simulink model "Lab7"  (R2021b)
settings: Solver=VariableStepAuto  StartTime=0.0  StopTime=T  RelTol=1e-3
values from neighbouring files (symbols this model uses):
  a = 1/( 2/norm(r0) - dot(v0,v0)/mu_E )    [Excercise1_2223.m]    (also in Excercise2_2223.m; Lab08_script.m = 42164; Lab7_script.m = 16733.65; Lab7_scriptscalar.m = 16733.65)
  A0 = eye(3)    [Lab08_script.m]    (also in Lab7_script.m; Lab7_scriptscalar.m; Lab_GG.m)
  Area_mb = diag([A1 A2 A3 A4 A5 A6])    [Lab08_script.m]    (also in Lab7_script.m)
  e = horizonsresults(:,2)    [Ex3-5.m]    (also in Excercise1_2223.m = 1/mu_E*cross(v,h)-r./vecnorm(r,2,2); Lab08_script.m = 0; Lab7_script.m = 0.1976; Lab7_scriptscalar.m = 0.1976)
  epsilon = (vecnorm(v,2,2)).^2/2-mu_E./vecnorm(r,2,2)    [Excercise1_2223.m]    (also in Lab08_script.m = deg2rad(23.45); Lab7_script.m = deg2rad(23.45); Lab7_scriptscalar.m = deg2rad(23.45))
  I = [Ix 0 0; 0 Iy 0; 0 0 Iz]    [Lab08_script.m]    (also in Lab7_script.m; Lab7_scriptscalar.m; Lab_GG.m)
  i = horizonsresults(:,3)    [Ex3-5.m]    (also in Lab08_script.m = deg2rad(0); Lab7_script.m = deg2rad(60); Lab7_scriptscalar.m = deg2rad(60); ex3_Lambert.m = kep_arr_M(3))
  I_inv = inv(I)    [Lab08_script.m]    (also in Lab7_script.m; Lab7_scriptscalar.m; Lab_GG.m)
  n = 10    [Chapter3.m]    (also in Lab08_script.m = sqrt(mu_E/(a^3)); Lab7_script.m = sqrt(mu_E/(a^3)); Lab7_scriptscalar.m = sqrt(mu_E/(a^3)); Lab_GG.m = sqrt(mu_E/( R_E+r_orbit)^3))
  N_b_mb = [n1'; n2'; n3'; n4'; n5'; n6']    [Lab08_script.m]    (also in Lab7_script.m)
  n_sun = 2*pi/T_sun    (= 1.99238499086e-07)    [Lab08_script.m]    (also in Lab7_script.m; Lab7_scriptscalar.m)
  P = Fe/c    (= 4.52666666667e-06)    [Lab08_script.m]    (also in Lab7_script.m; Lab7_scriptscalar.m)
  rho_d_mb = 0.1    [Lab08_script.m]    (also in Lab7_script.m; Lab7_scriptscalar.m)
  rho_s_mb = 0.5    [Lab08_script.m]    (also in Lab7_script.m; Lab7_scriptscalar.m)
  Rs = astroConstants(2)    [Lab08_script.m]    (also in Lab7_script.m; Lab7_scriptscalar.m)
  theta0 = deg2rad(0)    [Lab08_script.m]    (also in Lab7_script.m = deg2rad(230); Lab7_scriptscalar.m = deg2rad(230))
  v1 = [Y1(:,4) Y1(:,5) Y1(:,6)]    [Excercise2_2223.m]    (also in Lab08_script.m = [0 1 -1]'; Lab7_script.m = [0 1 -1]'; Lab7_scriptscalar.m = [0 1 -1]'; Lab_GG.m = [0 1 -1]')
  v2 = [Y2(:,4) Y2(:,5) Y2(:,6)]    [Excercise2_2223.m]    (also in Lab08_script.m = [-1 0 1]'; Lab7_script.m = [-1 0 1]'; Lab7_scriptscalar.m = [-1 0 1]'; Lab_GG.m = [-1 0 1]')
  v3 = [1 -1 0]'    [Lab08_script.m]    (also in Lab7_script.m; Lab7_scriptscalar.m; Lab_GG.m)
  w_0 = [wx_0 wy_0 wz_0]'    [Lab08_script.m]    (also in Lab7_script.m; Lab7_scriptscalar.m; Lab_GG.m)
libraries: matrix_library x1
settings Model: Creator=sferl  LastModifiedBy=sferl

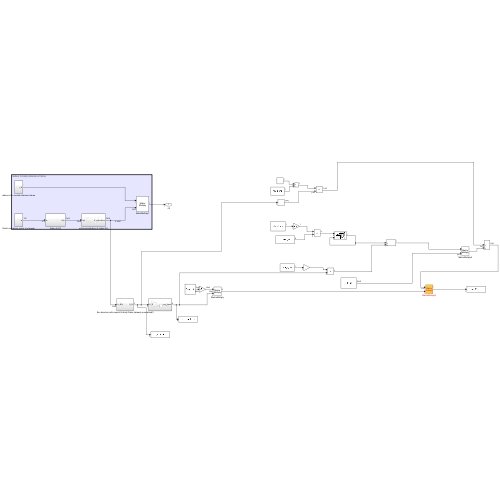
[thumbnail: Simulink's stored preview of the top-level diagram]
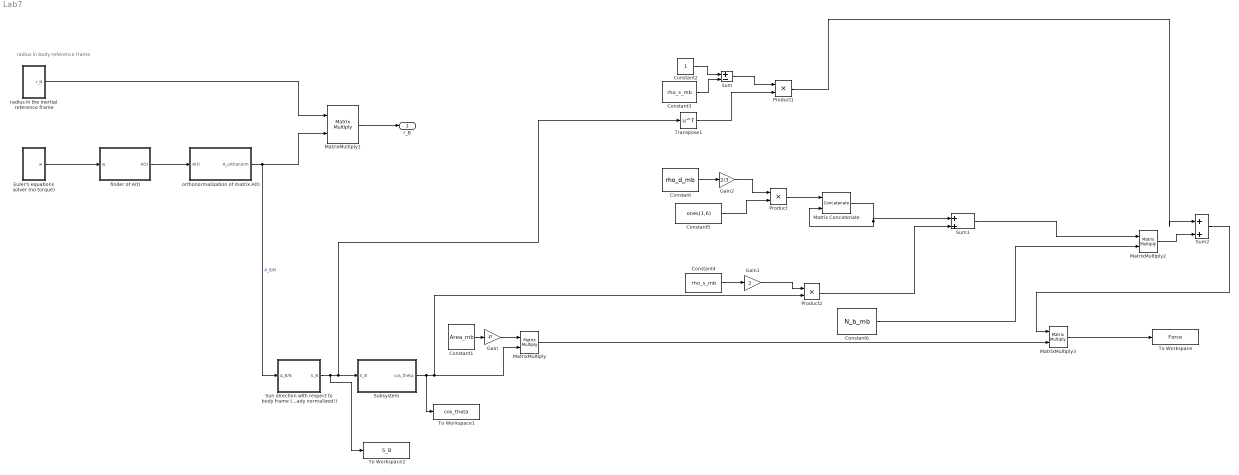
== system Lab7 ==
  note: radius in body reference frame
  Constant : Constant  Value=rho_d_mb
  Constant1 : Constant  Value=Area_mb
  Constant2 : Constant
  Constant3 : Constant  Value=rho_s_mb
  Constant4 : Constant  Value=rho_s_mb
  Constant5 : Constant  Value=ones(1,6)
  Constant6 : Constant  Value=N_b_mb
  Euler's equations solver (no torque) : Subsystem
  Gain : Gain  Gain=-P
  Gain1 : Gain  Gain=2
  Gain2 : Gain  Gain=2/3
  Matrix Concatenate : Concatenate  Mode=Multidimensional array
  MatrixMultiply{,1..3} (4 alike) : Product  Multiplication=Matrix(*)
  Product : Product
  Product1 : Product
  Product2 : Product
  Subsystem : Subsystem
  Sum : Sum  Inputs=+-
  Sum1 : Sum  Inputs=|++
  Sum2 : Sum  Inputs=|++
  Sun direction with respect to body frame (already normalized!) : Subsystem
  To Workspace : ToWorkspace  VariableName=Force  SaveFormat=Timeseries  SampleTime=-1
  To Workspace1 : ToWorkspace  VariableName=cos_theta  SampleTime=-1
  To Workspace2 : ToWorkspace  VariableName=S_B  SampleTime=-1
  Transpose1 : Math  Operator=transpose  SaturateOnIntegerOverflow=on
  finder of A(t) : Subsystem
  orthonormalization of matrix A(t) : Subsystem
  radius in the inertial reference frame : Subsystem
  r_B : Outport
  wires:
  MatrixMultiply1/1 -> r_B/1
  radius in the inertial reference frame/1(r_N) -> MatrixMultiply1/1
  finder of A(t)/1(A(t)) -> orthonormalization of matrix A(t)/1(A(t))
  orthonormalization of matrix A(t)/1(A_orthonorm) -> Sun direction with respect to body frame (already normalized!)/1(A_B/N), MatrixMultiply1/2  "A_B/N"
  Euler's equations solver (no torque)/1(w) -> finder of A(t)/1(w)
  Constant1/1 -> Gain/1
  Gain/1 -> MatrixMultiply/1
  Subsystem/1(cos_theta) -> To Workspace1/1, MatrixMultiply/2, Product2/2
  Sun direction with respect to body frame (already normalized!)/1(S_B) -> To Workspace2/1, Transpose1/1, Subsystem/1(S_B)
  Constant2/1 -> Sum/1
  Constant3/1 -> Sum/2
  Sum/1 -> Product1/1
  Constant4/1 -> Gain1/1
  Gain1/1 -> Product2/1
  Product2/1 -> Sum1/2
  Constant6/1 -> MatrixMultiply2/2
  MatrixMultiply2/1 -> Sum2/2
  Product1/1 -> Sum2/1
  MatrixMultiply/1 -> MatrixMultiply3/2
  Sum2/1 -> MatrixMultiply3/1
  MatrixMultiply3/1 -> To Workspace/1
  Transpose1/1 -> Product1/2
  Constant/1 -> Gain2/1
  Gain2/1 -> Product/1
  Constant5/1 -> Product/2
  Product/1 -> Matrix Concatenate/1
  Matrix Concatenate/1 -> Matrix Concatenate/2, Sum1/1
  Sum1/1 -> MatrixMultiply2/1

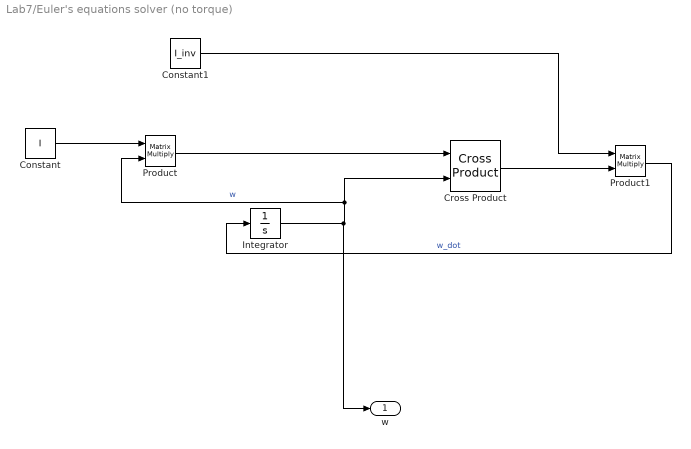
== system Lab7/Euler's equations solver (no torque) ==
  Constant : Constant  Value=I  VectorParams1D=off
  Constant1 : Constant  Value=I_inv  VectorParams1D=off
  Cross Product : matrix_library/Cross Product
      settings: SourceProductBaseCode=SL
  Integrator : Integrator  InitialCondition=w_0
  Product : Product  Multiplication=Matrix(*)
  Product1 : Product  Multiplication=Matrix(*)
  w : Outport
  wires:
  Product/1 -> Cross Product/1
  Constant/1 -> Product/1
  Constant1/1 -> Product1/1
  Cross Product/1 -> Product1/2
  Integrator/1 -> w/1, Cross Product/2, Product/2  "w"
  Product1/1 -> Integrator/1  "w_dot"

== system Lab7/Subsystem ==
  S_B : Inport
  Constant : Constant  Value=N_b_mb
  MatrixMultiply : Product  Multiplication=Matrix(*)
  cos_theta : Outport
  wires:
  Constant/1 -> MatrixMultiply/1
  MatrixMultiply/1 -> cos_theta/1
  S_B/1 -> MatrixMultiply/2

== system Lab7/Sun direction with respect to body frame (already normalized!) ==
  A_B/N : Inport
  Constant7 : Constant  Value=1/Rs
  MatrixMultiply : Product  Multiplication=Matrix(*)
  Product5 : Product
  S_N : Subsystem
  S_B : Outport
  wires:
  S_N/1(Out1) -> MatrixMultiply/2
  A_B/N/1 -> MatrixMultiply/1
  Constant7/1 -> Product5/1
  MatrixMultiply/1 -> Product5/2
  Product5/1 -> S_B/1

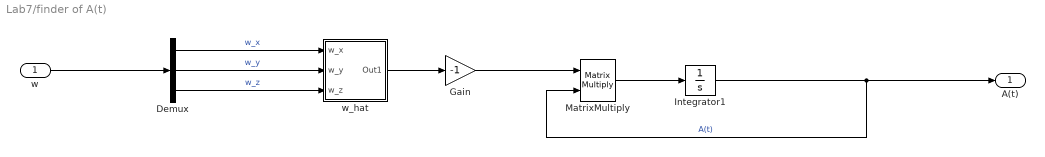
== system Lab7/finder of A(t) ==
  w : Inport
  Demux : Demux  Outputs=3
  Gain : Gain  Gain=-1
  Integrator1 : Integrator  InitialCondition=A0
  MatrixMultiply : Product  Multiplication=Matrix(*)
  w_hat : Subsystem
  A(t) : Outport
  wires:
  w/1 -> Demux/1
  Gain/1 -> MatrixMultiply/1
  Integrator1/1 -> A(t)/1, MatrixMultiply/2  "A(t)"
  w_hat/1(Out1) -> Gain/1
  Demux/3 -> w_hat/3(w_z)  "w_z"
  Demux/2 -> w_hat/2(w_y)  "w_y"
  Demux/1 -> w_hat/1(w_x)  "w_x"
  MatrixMultiply/1 -> Integrator1/1

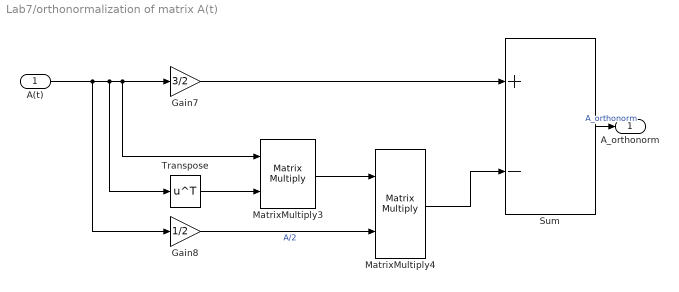
== system Lab7/orthonormalization of matrix A(t) ==
  A(t) : Inport
  Gain7 : Gain  Gain=3/2
  Gain8 : Gain  Gain=1/2
  MatrixMultiply3 : Product  Multiplication=Matrix(*)
  MatrixMultiply4 : Product  Multiplication=Matrix(*)
  Sum : Sum  Inputs=+-
  Transpose : Math  Operator=transpose  SaturateOnIntegerOverflow=on
  A_orthonorm : Outport
  wires:
  Transpose/1 -> MatrixMultiply3/2
  MatrixMultiply4/1 -> Sum/2
  MatrixMultiply3/1 -> MatrixMultiply4/1
  Gain7/1 -> Sum/1
  Gain8/1 -> MatrixMultiply4/2  "A/2"
  A(t)/1 -> Gain8/1, Transpose/1, MatrixMultiply3/1, Gain7/1
  Sum/1 -> A_orthonorm/1  "A_orthonorm"

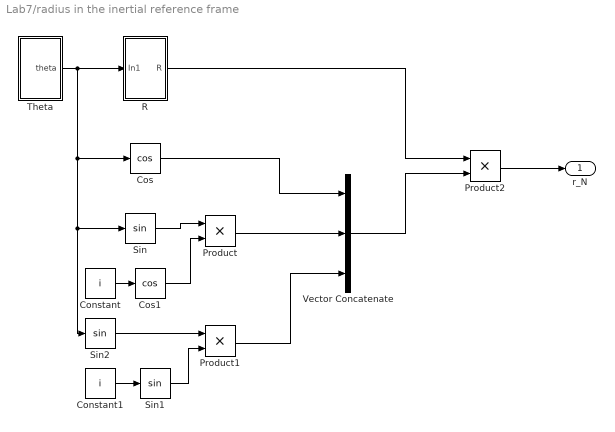
== system Lab7/radius in the inertial reference frame ==
  Constant : Constant  Value=i
  Constant1 : Constant  Value=i
  Cos : Trigonometry  Operator=cos
  Cos1 : Trigonometry  Operator=cos
  Product : Product
  Product1 : Product
  Product2 : Product
  R : Subsystem
  Sin : Trigonometry
  Sin1 : Trigonometry
  Sin2 : Trigonometry
  Theta : Subsystem
  Vector Concatenate : Concatenate  NumInputs=3
  r_N : Outport
  wires:
  Cos/1 -> Vector Concatenate/1
  Theta/1(theta) -> Sin2/1, Sin/1, Cos/1, R/1(In1)
  Constant/1 -> Cos1/1
  Product1/1 -> Vector Concatenate/3
  Sin1/1 -> Product1/2
  Cos1/1 -> Product/2
  R/1(R) -> Product2/1
  Product/1 -> Vector Concatenate/2
  Vector Concatenate/1 -> Product2/2
  Constant1/1 -> Sin1/1
  Sin/1 -> Product/1
  Sin2/1 -> Product1/1
  Product2/1 -> r_N/1

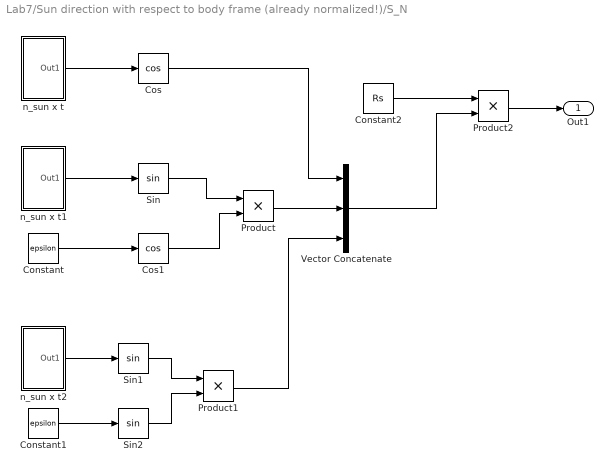
== system Lab7/Sun direction with respect to body frame (already normalized!)/S_N ==
  Constant : Constant  Value=epsilon
  Constant1 : Constant  Value=epsilon
  Constant2 : Constant  Value=Rs
  Cos : Trigonometry  Operator=cos
  Cos1 : Trigonometry  Operator=cos
  Product : Product
  Product1 : Product
  Product2 : Product
  Sin : Trigonometry
  Sin1 : Trigonometry
  Sin2 : Trigonometry
  Vector Concatenate : Concatenate  NumInputs=3
  n_sun x t : Subsystem
  n_sun x t1 : Subsystem
  n_sun x t2 : Subsystem
  Out1 : Outport
  wires:
  n_sun x t2/1(Out1) -> Sin1/1
  Vector Concatenate/1 -> Product2/2
  Sin2/1 -> Product1/2
  Sin/1 -> Product/1
  n_sun x t1/1(Out1) -> Sin/1
  Product1/1 -> Vector Concatenate/3
  Constant2/1 -> Product2/1
  Cos/1 -> Vector Concatenate/1
  Cos1/1 -> Product/2
  Product/1 -> Vector Concatenate/2
  n_sun x t/1(Out1) -> Cos/1
  Constant1/1 -> Sin2/1
  Sin1/1 -> Product1/1
  Constant/1 -> Cos1/1
  Product2/1 -> Out1/1

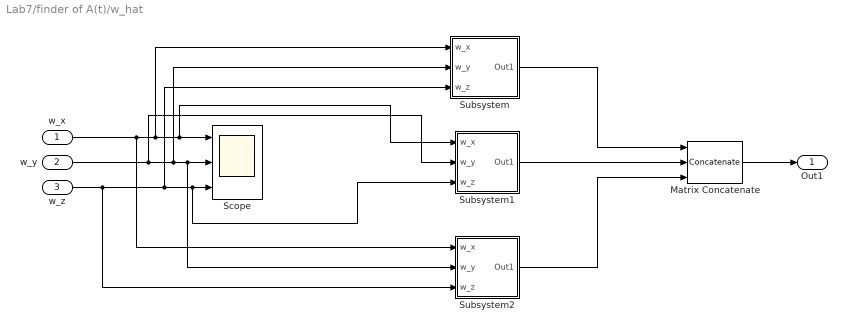
== system Lab7/finder of A(t)/w_hat ==
  w_x : Inport
  w_y : Inport  Port=2
  w_z : Inport  Port=3
  Matrix Concatenate : Concatenate  NumInputs=3  Mode=Multidimensional array  ConcatenateDimension=2
  Scope : Scope  NumInputPorts=3
  Subsystem : Subsystem
  Subsystem1 : Subsystem
  Subsystem2 : Subsystem
  Out1 : Outport
  wires:
  w_y/1 -> Subsystem1/2(w_y), Subsystem/2(w_y), Subsystem2/2(w_y), Scope/2
  w_z/1 -> Subsystem2/3(w_z), Subsystem/3(w_z), Subsystem1/3(w_z), Scope/3
  w_x/1 -> Subsystem2/1(w_x), Subsystem/1(w_x), Subsystem1/1(w_x), Scope/1
  Subsystem2/1(Out1) -> Matrix Concatenate/3
  Subsystem1/1(Out1) -> Matrix Concatenate/2
  Subsystem/1(Out1) -> Matrix Concatenate/1
  Matrix Concatenate/1 -> Out1/1

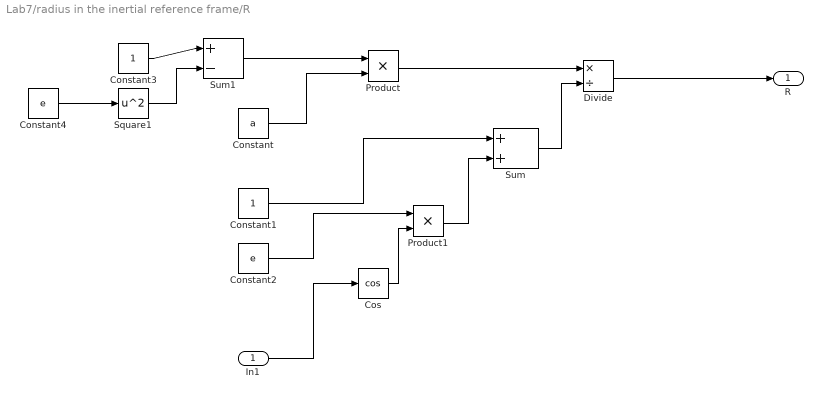
== system Lab7/radius in the inertial reference frame/R ==
  In1 : Inport
  Constant : Constant  Value=a
  Constant1 : Constant
  Constant2 : Constant  Value=e
  Constant3 : Constant
  Constant4 : Constant  Value=e
  Cos : Trigonometry  Operator=cos
  Divide : Product  Inputs=*/
  Product : Product
  Product1 : Product
  Square1 : Math  Operator=square  SaturateOnIntegerOverflow=on
  Sum : Sum  Inputs=|++
  Sum1 : Sum  Inputs=|+-
  R : Outport
  wires:
  Sum/1 -> Divide/2
  Constant1/1 -> Sum/1
  Square1/1 -> Sum1/2
  Product1/1 -> Sum/2
  Constant2/1 -> Product1/1
  Constant/1 -> Product/2
  Divide/1 -> R/1
  Cos/1 -> Product1/2
  Sum1/1 -> Product/1
  In1/1 -> Cos/1
  Constant4/1 -> Square1/1
  Constant3/1 -> Sum1/1
  Product/1 -> Divide/1

== system Lab7/radius in the inertial reference frame/Theta ==
  Denominator : Subsystem
  Divide : Product  Inputs=*/
  Integrator : Integrator  InitialCondition=theta0
  Numerator : Subsystem
  To Workspace : ToWorkspace  VariableName=theta  SampleTime=-1
  theta : Outport
  wires:
  Numerator/1(Out1) -> Divide/1
  Denominator/1(Out1) -> Divide/2
  Integrator/1 -> theta/1, Numerator/1(In1), To Workspace/1
  Divide/1 -> Integrator/1

== system Lab7/Sun direction with respect to body frame (already normalized!)/S_N/n_sun x t ==
  Clock : Clock
  Constant : Constant  Value=n_sun
  Product : Product
  Out1 : Outport
  wires:
  Constant/1 -> Product/1
  Clock/1 -> Product/2
  Product/1 -> Out1/1

== system Lab7/Sun direction with respect to body frame (already normalized!)/S_N/n_sun x t1 ==
  Clock : Clock
  Constant : Constant  Value=n_sun
  Product : Product
  Out1 : Outport
  wires:
  Product/1 -> Out1/1
  Clock/1 -> Product/2
  Constant/1 -> Product/1

== system Lab7/Sun direction with respect to body frame (already normalized!)/S_N/n_sun x t2 ==
  Clock : Clock
  Constant : Constant  Value=n_sun
  Product : Product
  Out1 : Outport
  wires:
  Constant/1 -> Product/1
  Clock/1 -> Product/2
  Product/1 -> Out1/1

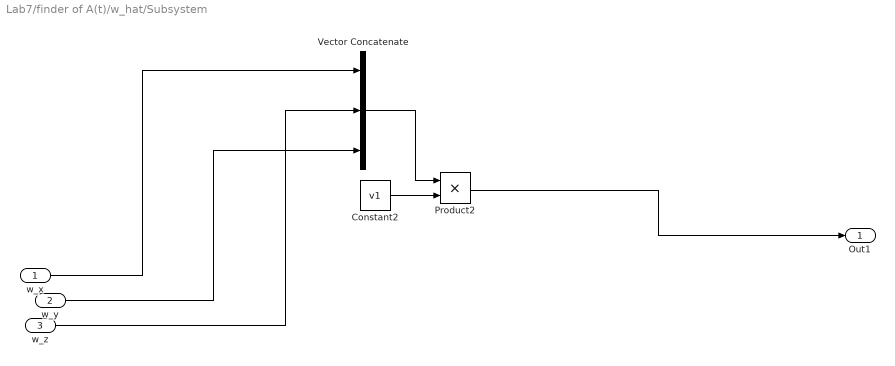
== system Lab7/finder of A(t)/w_hat/Subsystem ==
  w_x : Inport
  w_y : Inport  Port=2
  w_z : Inport  Port=3
  Constant2 : Constant  Value=v1
  Product2 : Product
  Vector Concatenate : Concatenate  NumInputs=3
  Out1 : Outport
  wires:
  Product2/1 -> Out1/1
  Vector Concatenate/1 -> Product2/1
  Constant2/1 -> Product2/2
  w_x/1 -> Vector Concatenate/1
  w_z/1 -> Vector Concatenate/2
  w_y/1 -> Vector Concatenate/3

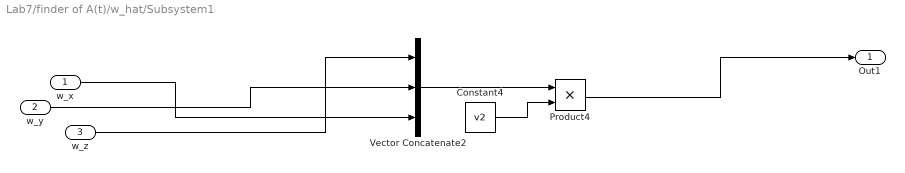
== system Lab7/finder of A(t)/w_hat/Subsystem1 ==
  w_x : Inport
  w_y : Inport  Port=2
  w_z : Inport  Port=3
  Constant4 : Constant  Value=v2
  Product4 : Product
  Vector Concatenate2 : Concatenate  NumInputs=3
  Out1 : Outport
  wires:
  Constant4/1 -> Product4/2
  Vector Concatenate2/1 -> Product4/1
  Product4/1 -> Out1/1
  w_x/1 -> Vector Concatenate2/3
  w_y/1 -> Vector Concatenate2/2
  w_z/1 -> Vector Concatenate2/1

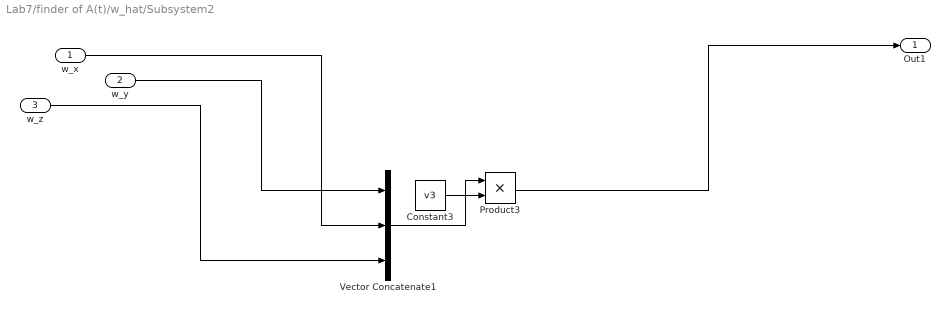
== system Lab7/finder of A(t)/w_hat/Subsystem2 ==
  w_x : Inport
  w_y : Inport  Port=2
  w_z : Inport  Port=3
  Constant3 : Constant  Value=v3
  Product3 : Product
  Vector Concatenate1 : Concatenate  NumInputs=3
  Out1 : Outport
  wires:
  Product3/1 -> Out1/1
  Constant3/1 -> Product3/2
  w_y/1 -> Vector Concatenate1/1
  Vector Concatenate1/1 -> Product3/1
  w_x/1 -> Vector Concatenate1/2
  w_z/1 -> Vector Concatenate1/3

== system Lab7/radius in the inertial reference frame/Theta/Denominator ==
  Constant3 : Constant
  Constant4 : Constant  Value=e
  Constant5 : Constant  Value=3/2
  Power : Math  Operator=pow  SaturateOnIntegerOverflow=on
  Square1 : Math  Operator=square  SaturateOnIntegerOverflow=on
  Sum1 : Sum  Inputs=|+-
  Out1 : Outport
  wires:
  Constant3/1 -> Sum1/1
  Constant4/1 -> Square1/1
  Sum1/1 -> Power/1
  Square1/1 -> Sum1/2
  Constant5/1 -> Power/2
  Power/1 -> Out1/1

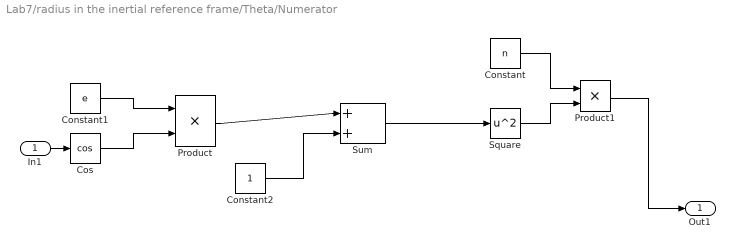
== system Lab7/radius in the inertial reference frame/Theta/Numerator ==
  In1 : Inport
  Constant : Constant  Value=n
  Constant1 : Constant  Value=e
  Constant2 : Constant
  Cos : Trigonometry  Operator=cos
  Product : Product
  Product1 : Product
  Square : Math  Operator=square  SaturateOnIntegerOverflow=on
  Sum : Sum  Inputs=|++
  Out1 : Outport
  wires:
  Constant2/1 -> Sum/2
  Sum/1 -> Square/1
  In1/1 -> Cos/1
  Constant1/1 -> Product/1
  Constant/1 -> Product1/1
  Cos/1 -> Product/2
  Product/1 -> Sum/1
  Square/1 -> Product1/2
  Product1/1 -> Out1/1
